simulink model "Pwm_Scalar_control"  (R2021b)
settings: Solver=FixedStepDiscrete  StartTime=0.0  StopTime=inf  RelTol=1e-3  EnableMultiTasking=on
undefined symbols (not defined in the file or in its folder): Down, Up
libraries: c280xlib x4, simulink x3, c2833xlib x1, c2000lib x1
settings Model: Creator=The MathWorks, Inc.  LastModifiedBy=pawan
settings SolverCC: AlgebraicLoopSolver=TrustRegion
settings DataIOCC: LimitDataPoints=on  SaveFormat=Array  SaveOutput=off  SaveTime=off  ReturnWorkspaceOutputs=off
settings OptimizationCC: ExpressionDepthLimit=2147483647  InitFltsAndDblsToZero=on  LifeSpan=inf  MaxStackSize=64  EfficientTunableParamExpr=on
settings DebuggingCC: UnderspecifiedInitializationDetection=Classic  MergeDetectMultiDrivingBlocksExec=none  SignalResolutionControl=TryResolveAllWithWarning  InheritedTsInSrcMsg=none  MultiTaskDSMMsg=warning  MultiTaskCondExecSysMsg=none  FcnCallInpInsideContextMsg=warning  AllowSymbolicDim=off  StateNameClashWarn=warning  SFUnexpectedBacktrackingDiag=warning  SFNoUnconditionalDefaultTransitionDiag=warning  SFExecutionAtInitializationDiag=none  SFMachineParentedDataDiag=warning  ArithmeticOperatorsInVariantConditions=warning
settings HardwareCC: ProdBitPerChar=16  ProdBitPerInt=16  ProdBitPerPointer=32  ProdBitPerSizeT=32  ProdBitPerPtrDiffT=32  ProdLargestAtomicInteger=Integer  ProdLargestAtomicFloat=None  ProdWordSize=16  ProdHWDeviceType=Texas Instruments->C2000  TargetBitPerChar=16  TargetBitPerInt=16  TargetBitPerPointer=16  TargetLargestAtomicInteger=Integer  TargetIntDivRoundTo=Zero  TargetEndianess=LittleEndian  TargetWordSize=16  TargetHWDeviceType=Texas Instruments->C2000  ProdEqTarget=off
settings ModelReferenceCC: PropagateSignalLabelsOutOfModel=off
settings SFSimCC: SimUseLocalCustomCode=off  MATLABDynamicMemAlloc=off  CustomCodeUndefinedFunction=UseInterfaceOnly
settings RTWCC: Description=Embedded Coder  SystemTargetFile=ert.tlc  HardwareBoard=TI Delfino F2833x  TemplateMakefile=ert_default_tmf  PostCodeGenCommand=; codertarget.postCodeGenHookCommand(h)  RTWUseLocalCustomCode=off  Toolchain=Texas Instruments Code Composer Studio (C2000)
settings CodeAppCC: IgnoreCustomStorageClasses=off  CustomSymbolStrType=$N$R$M  StateflowObjectComments=on  InternalIdentifier=Classic
settings ERTTargetCC: MultiwordLength=2048  ParMdlRefBuildCompliant=off  CompOptLevelCompliant=off  ConcurrentExecutionCompliant=off  CPPClassGenCompliant=off  ExtModeTransport=4  ExtModeStaticAlloc=on  ExtModeStaticAllocSize=2048  ExtModeMexFile=ext_xcp  ExtModeIntrfLevel=Level2 - Open  ConvertIfToSwitch=off  SuppressUnreachableDefaultCases=off
settings ConfigComp: CovMetricSettings=dw  CovSaveCumulativeToWorkspaceVar=on  CovSaveSingleToWorkspaceVar=on  CovExternalEMLEnable=off  CovSFcnEnable=off

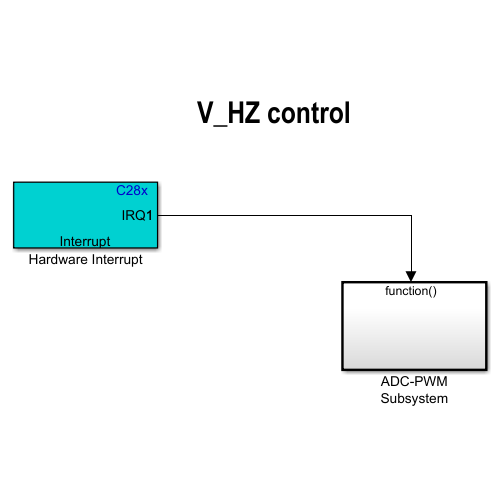
[thumbnail: Simulink's stored preview of the top-level diagram]
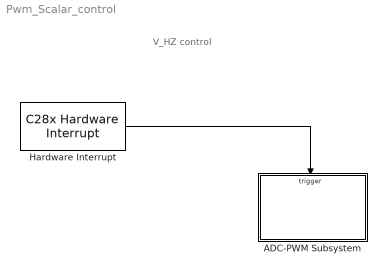
== system Pwm_Scalar_control ==
  note: V_HZ control
  ADC-PWM Subsystem : Subsystem  TreatAsAtomicUnit=on
  Hardware Interrupt : c2000lib/Scheduling/C28x Hardware Interrupt  irqnumbers=[1]  pienumbers=[1]  irqpriorities=[30]  irqpreempts=[0]  showinput=off  dspchiptype=C280X
      settings: SourceProductBaseCode=TIC2000
  wires:
  Hardware Interrupt/1 -> ADC-PWM Subsystem/Trigger

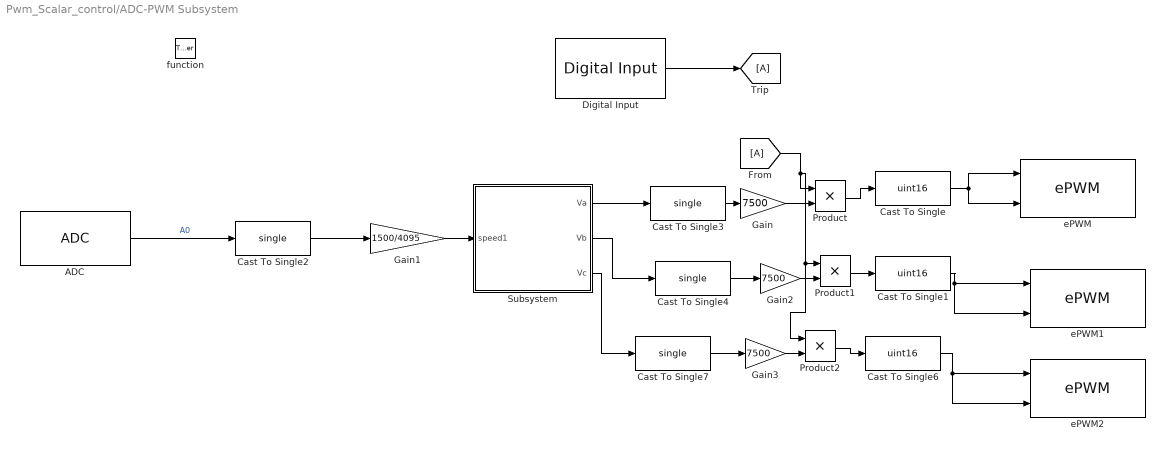
== system Pwm_Scalar_control/ADC-PWM Subsystem ==
  function : TriggerPort  TriggerType=function-call  VariantControl=Variant
  ADC : c280xlib/ADC  useModule=A  useMode=Sequential  sourceSOC=Software  sourceSOC1=ePWMxA  sourceSOC2=ePWMxB  xint2_ADCSOC=31  Ts=-1  dType=single  postInterrupt=on  numConversionsSingle=1  numConversionsDouble=1  conv0=ADCINA0  conv1=ADCINA1  conv2=ADCINA2  conv3=ADCINA3  conv4=ADCINA4  conv5=ADCINA5  conv6=ADCINA6  conv7=ADCINA7  conv8=ADCINB0  conv9=ADCINB1  conv10=ADCINB2  conv11=ADCINB3  conv12=ADCINB4  conv13=ADCINB5  conv14=ADCINB6  conv15=ADCINB7  convAB0=ADCINA0 and ADCINB0  convAB1=ADCINA1 and ADCINB1  convAB2=ADCINA2 and ADCINB2  convAB3=ADCINA3 and ADCINB3  convAB4=ADCINA4 and ADCINB4  convAB5=ADCINA5 and ADCINB5  convAB6=ADCINA6 and ADCINB6  convAB7=ADCINA7 and ADCINB7  convA0=ADCINA0  convA1=ADCINA1  convA2=ADCINA2  convA3=ADCINA3  convA4=ADCINA4  convA5=ADCINA5  convA6=ADCINA6  convA7=ADCINA7  convB0=ADCINB0  convB1=ADCINB1  convB2=ADCINB2  convB3=ADCINB3  convB4=ADCINB4  convB5=ADCINB5  convB6=ADCINB6  convB7=ADCINB7  c28xmultiPort=off  endma=off  chdma=1
      settings: SourceProductBaseCode=TIC2000
  Cast To Single : DataTypeConversion  OutDataTypeStr=uint16
  Cast To Single1 : DataTypeConversion  OutDataTypeStr=uint16
  Cast To Single{2..4,7} (4 alike) : DataTypeConversion  OutDataTypeStr=single  LockScale=on
  Cast To Single6 : DataTypeConversion  OutDataTypeStr=uint16
  Digital Input : c2833xlib/Digital Input  GPIO_Number=GPIO56~GPIO63  GPIO_Bit0=off  GPIO_Bit1=off  GPIO_Bit2=off  GPIO_Bit3=off  GPIO_Bit4=on  GPIO_Bit5=off  GPIO_Bit6=off  GPIO_Bit7=off  sampleTime=-1  dataType=auto  GPIO_Bit0_Qualification=Sync to SYSCLKOUT  GPIO_Bit1_Qualification=Sync to SYSCLKOUT  GPIO_Bit2_Qualification=Sync to SYSCLKOUT  GPIO_Bit3_Qualification=Sync to SYSCLKOUT  GPIO_Bit4_Qualification=Sync to SYSCLKOUT  GPIO_Bit5_Qualification=Sync to SYSCLKOUT  GPIO_Bit6_Qualification=Sync to SYSCLKOUT  GPIO_Bit7_Qualification=Sync to SYSCLKOUT  Qualification_Period=-1
      settings: SourceProductBaseCode=TIC2000
  Gain : Gain  Gain=7500
  Gain1 : Gain  Gain=1500/4095  OutDataTypeStr=Inherit: Same as input  ParamDataTypeStr=Inherit: Same as input
  Gain2 : Gain  Gain=7500
  Gain3 : Gain  Gain=7500
  Product : Product
  Product1 : Product
  Product2 : Product
  Subsystem : Subsystem
  ePWM : c280xlib/ePWM  checkMode=off  useModule=ePWM2  periodUnits=Clock cycles  timerSource=Specify via dialog  timerPeriod_clk=7500  timerPeriod_sec=0.0001  tbshadow=Counter equals to zero  countingMode=Up-Down  phaseActiveEnable=Disable  phaseDirection=Count down after sync  phaseActive=0  synchronizationEnable=off  synchronizationOption=Disable  clockPrescale=1  HSclockPrescale=1  ePWMxAStatus=on  CMPAUnits=Clock cycles  CMPASource=Input port  CMPAValue_per=0  CMPAValue_clk=0  enCMPAshadow=Counter equals to zero  ePWMxAactionLogic1=Do nothing  ePWMxAactionLogic2=Do nothing  ePWMxAactionLogic3=Clear  ePWMxAactionLogic4=Set  ePWMxAactionLogic5=Do nothing  ePWMxAactionLogic6=Do nothing  ePWMxALoadMode=Load on counter equals to zero (CTR=Zero)  ePWMxACSFenable=off  ePWMxACSFvalue=Forcing disable  ePWMxASFreload=Zero  enHRPWM=off  HRPWM_LoadMode=Counter equals to zero (CTR=ZERO)  HRPWM_CTLMode=Phase control mode  HRPWM_EDGMode=Both edge  enSFO=on  ePWMxBStatus=off  CMPBUnits=Percentages  CMPBSource=Input port  CMPBValue_per=0  CMPBValue_clk=0  enCMPBshadow=Counter equals to zero  ePWMxBactionLogic1=Do nothing  ePWMxBactionLogic2=Do nothing  ePWMxBactionLogic3=Do nothing  ePWMxBactionLogic4=Do nothing  ePWMxBactionLogic5=Clear  ePWMxBactionLogic6=Set  ePWMxBLoadMode=Load on counter equals to zero (CTR=Zero)  ePWMxBCSFenable=off  ePWMxBCSFvalue=Forcing disable  ePWMxBSFreload=Zero  enableDBePWMxA=on  enableDBePWMxB=on  DBpolarity=Active high complementary (AHC)  DBedgeDelay=Positive  DBSource_ePWMxA=ePWMxA  DBSource_ePWMxB=ePWMxA  DBperiodSource=Specify via dialog  REDperiod=350  FEDperiod=350  adcstartModuleA=on  adcrequestEventA=First event  adcstartEventA=Counter equals to period (CTR=PRD)  adcstartModuleB=off  adcrequestEventB=First event  adcstartEventB=Counter equals to zero (CTR=Zero)  intEn=off  intPrd=First event  intSel=Counter equals to zero (CTR=Zero)  chopperEnable=off  chopperFrequency=1  chopperFirstwidth=1  chopperDuty=12.5%  tripZonesource=Specify via dialog  tzselOSHT1=off  tzselOSHT2=off  tzselOSHT3=off  tzselOSHT4=off  tzselOSHT5=off  tzselOSHT6=off  tzselCBC1=off  tzselCBC2=off  tzselCBC3=off  tzselCBC4=off  tzselCBC5=off  tzselCBC6=off  enTzOstIntr=off  enTzCbcIntr=off  ePWMxAforced=Low  ePWMxBforced=Low  timerPeriod=-1  ePWMxAValue=1  ePWMxBValue=0  tripZoneoption=One-shot trip (OSHT)
      settings: SourceProductBaseCode=TIC2000
  ePWM1 : c280xlib/ePWM  checkMode=off  useModule=ePWM3  periodUnits=Clock cycles  timerSource=Specify via dialog  timerPeriod_clk=7500  timerPeriod_sec=0.0001  tbshadow=Counter equals to zero  countingMode=Up-Down  phaseActiveEnable=Disable  phaseDirection=Count down after sync  phaseActive=0  synchronizationEnable=off  synchronizationOption=Disable  clockPrescale=1  HSclockPrescale=1  ePWMxAStatus=on  CMPAUnits=Clock cycles  CMPASource=Input port  CMPAValue_per=0  CMPAValue_clk=0  enCMPAshadow=Counter equals to zero  ePWMxAactionLogic1=Do nothing  ePWMxAactionLogic2=Do nothing  ePWMxAactionLogic3=Clear  ePWMxAactionLogic4=Set  ePWMxAactionLogic5=Do nothing  ePWMxAactionLogic6=Do nothing  ePWMxALoadMode=Load on counter equals to zero (CTR=Zero)  ePWMxACSFenable=off  ePWMxACSFvalue=Forcing disable  ePWMxASFreload=Zero  enHRPWM=off  HRPWM_LoadMode=Counter equals to zero (CTR=ZERO)  HRPWM_CTLMode=Phase control mode  HRPWM_EDGMode=Both edge  enSFO=on  ePWMxBStatus=off  CMPBUnits=Percentages  CMPBSource=Input port  CMPBValue_per=0  CMPBValue_clk=0  enCMPBshadow=Counter equals to zero  ePWMxBactionLogic1=Do nothing  ePWMxBactionLogic2=Do nothing  ePWMxBactionLogic3=Do nothing  ePWMxBactionLogic4=Do nothing  ePWMxBactionLogic5=Clear  ePWMxBactionLogic6=Set  ePWMxBLoadMode=Load on counter equals to zero (CTR=Zero)  ePWMxBCSFenable=off  ePWMxBCSFvalue=Forcing disable  ePWMxBSFreload=Zero  enableDBePWMxA=on  enableDBePWMxB=on  DBpolarity=Active high complementary (AHC)  DBedgeDelay=Positive  DBSource_ePWMxA=ePWMxA  DBSource_ePWMxB=ePWMxA  DBperiodSource=Specify via dialog  REDperiod=350  FEDperiod=350  adcstartModuleA=on  adcrequestEventA=First event  adcstartEventA=Counter equals to period (CTR=PRD)  adcstartModuleB=off  adcrequestEventB=First event  adcstartEventB=Counter equals to zero (CTR=Zero)  intEn=off  intPrd=First event  intSel=Counter equals to zero (CTR=Zero)  chopperEnable=off  chopperFrequency=1  chopperFirstwidth=1  chopperDuty=12.5%  tripZonesource=Specify via dialog  tzselOSHT1=off  tzselOSHT2=off  tzselOSHT3=off  tzselOSHT4=off  tzselOSHT5=off  tzselOSHT6=off  tzselCBC1=off  tzselCBC2=off  tzselCBC3=off  tzselCBC4=off  tzselCBC5=off  tzselCBC6=off  enTzOstIntr=off  enTzCbcIntr=off  ePWMxAforced=Low  ePWMxBforced=Low  timerPeriod=-1  ePWMxAValue=1  ePWMxBValue=0  tripZoneoption=One-shot trip (OSHT)
      settings: SourceProductBaseCode=TIC2000
  ePWM2 : c280xlib/ePWM  checkMode=off  useModule=ePWM4  periodUnits=Clock cycles  timerSource=Specify via dialog  timerPeriod_clk=7500  timerPeriod_sec=0.0001  tbshadow=Counter equals to zero  countingMode=Up-Down  phaseActiveEnable=Disable  phaseDirection=Count down after sync  phaseActive=0  synchronizationEnable=off  synchronizationOption=Disable  clockPrescale=1  HSclockPrescale=1  ePWMxAStatus=on  CMPAUnits=Clock cycles  CMPASource=Input port  CMPAValue_per=0  CMPAValue_clk=0  enCMPAshadow=Counter equals to zero  ePWMxAactionLogic1=Do nothing  ePWMxAactionLogic2=Do nothing  ePWMxAactionLogic3=Clear  ePWMxAactionLogic4=Set  ePWMxAactionLogic5=Do nothing  ePWMxAactionLogic6=Do nothing  ePWMxALoadMode=Load on counter equals to zero (CTR=Zero)  ePWMxACSFenable=off  ePWMxACSFvalue=Forcing disable  ePWMxASFreload=Zero  enHRPWM=off  HRPWM_LoadMode=Counter equals to zero (CTR=ZERO)  HRPWM_CTLMode=Phase control mode  HRPWM_EDGMode=Both edge  enSFO=on  ePWMxBStatus=off  CMPBUnits=Percentages  CMPBSource=Input port  CMPBValue_per=0  CMPBValue_clk=0  enCMPBshadow=Counter equals to zero  ePWMxBactionLogic1=Do nothing  ePWMxBactionLogic2=Do nothing  ePWMxBactionLogic3=Do nothing  ePWMxBactionLogic4=Do nothing  ePWMxBactionLogic5=Clear  ePWMxBactionLogic6=Set  ePWMxBLoadMode=Load on counter equals to zero (CTR=Zero)  ePWMxBCSFenable=off  ePWMxBCSFvalue=Forcing disable  ePWMxBSFreload=Zero  enableDBePWMxA=on  enableDBePWMxB=on  DBpolarity=Active high complementary (AHC)  DBedgeDelay=Positive  DBSource_ePWMxA=ePWMxA  DBSource_ePWMxB=ePWMxA  DBperiodSource=Specify via dialog  REDperiod=350  FEDperiod=350  adcstartModuleA=on  adcrequestEventA=First event  adcstartEventA=Counter equals to period (CTR=PRD)  adcstartModuleB=off  adcrequestEventB=First event  adcstartEventB=Counter equals to zero (CTR=Zero)  intEn=off  intPrd=First event  intSel=Counter equals to zero (CTR=Zero)  chopperEnable=off  chopperFrequency=1  chopperFirstwidth=1  chopperDuty=12.5%  tripZonesource=Specify via dialog  tzselOSHT1=off  tzselOSHT2=off  tzselOSHT3=off  tzselOSHT4=off  tzselOSHT5=off  tzselOSHT6=off  tzselCBC1=off  tzselCBC2=off  tzselCBC3=off  tzselCBC4=off  tzselCBC5=off  tzselCBC6=off  enTzOstIntr=off  enTzCbcIntr=off  ePWMxAforced=Low  ePWMxBforced=Low  timerPeriod=-1  ePWMxAValue=1  ePWMxBValue=0  tripZoneoption=One-shot trip (OSHT)
      settings: SourceProductBaseCode=TIC2000
  wires:
  ADC/1 -> Cast To Single2/1  "A0"
  Gain1/1 -> Subsystem/1(speed1)
  Cast To Single2/1 -> Gain1/1
  Cast To Single3/1 -> Gain/1
  Cast To Single/1 -> ePWM/2, ePWM/1
  Cast To Single4/1 -> Gain2/1
  Cast To Single1/1 -> ePWM1/1, ePWM1/2
  Cast To Single7/1 -> Gain3/1
  Cast To Single6/1 -> ePWM2/1, ePWM2/2
  Subsystem/3(Vc) -> Cast To Single7/1
  Subsystem/2(Vb) -> Cast To Single4/1
  Subsystem/1(Va) -> Cast To Single3/1
  Gain/1 -> Product/2
  Product/1 -> Cast To Single/1
  Gain2/1 -> Product1/2
  Product1/1 -> Cast To Single1/1
  Product2/1 -> Cast To Single6/1
  Gain3/1 -> Product2/2
  Digital Input/1 -> [A]
  [A] -> Product2/1, Product1/1, Product/1

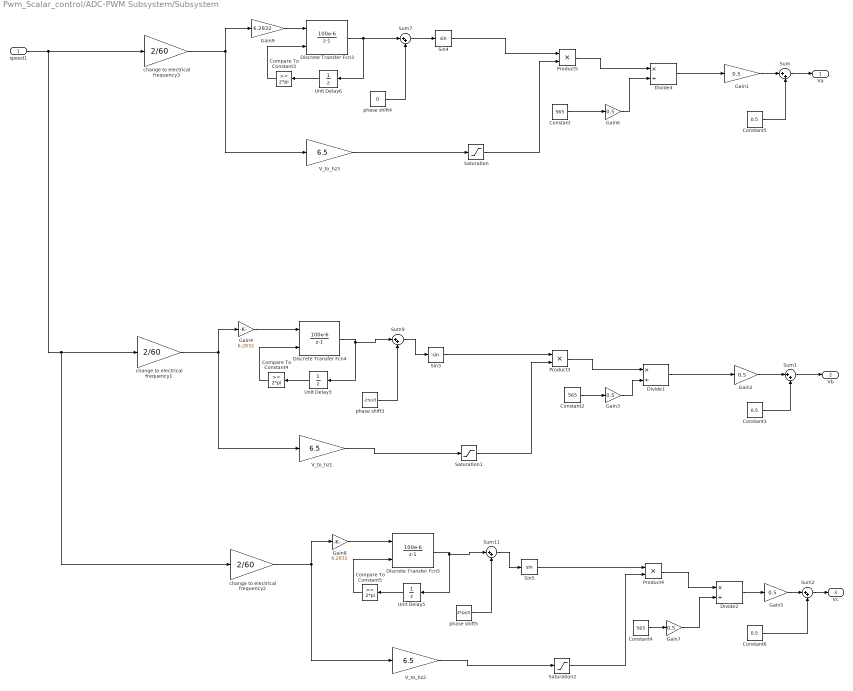
== system Pwm_Scalar_control/ADC-PWM Subsystem/Subsystem ==
  speed1 : Inport
  Compare To Constant3 : simulink/Logic and Bit Operations/Compare To Constant  relop=>=  const=2*pi  OutDataTypeStr=boolean
  Compare To Constant4 : simulink/Logic and Bit Operations/Compare To Constant  relop=>=  const=2*pi  OutDataTypeStr=boolean
  Compare To Constant5 : simulink/Logic and Bit Operations/Compare To Constant  relop=>=  const=2*pi  OutDataTypeStr=boolean
  Constant : Constant  Value=565
  Constant2 : Constant  Value=565
  Constant3 : Constant  Value=0.5  SampleTime=-1
  Constant4 : Constant  Value=565
  Constant5 : Constant  Value=0.5  SampleTime=-1
  Constant6 : Constant  Value=0.5  SampleTime=-1
  Discrete Transfer Fcn3 : DiscreteTransferFcn  Numerator=[100e-6]  Denominator=[1 -1]  ExternalReset=Rising
      settings: InputPortMap=u0,r7
  Discrete Transfer Fcn4 : DiscreteTransferFcn  Numerator=[100e-6]  Denominator=[1 -1]  ExternalReset=Rising
      settings: InputPortMap=u0,r7
  Discrete Transfer Fcn5 : DiscreteTransferFcn  Numerator=[100e-6]  Denominator=[1 -1]  ExternalReset=Rising
      settings: InputPortMap=u0,r7
  Divide1 : Product  Inputs=*/
  Divide2 : Product  Inputs=*/
  Divide4 : Product  Inputs=*/
  Gain{1..3,5..7} (6 alike) : Gain  Gain=0.5
  Gain4 : Gain  Gain=6.2832
  Gain8 : Gain  Gain=6.2832
  Gain9 : Gain  Gain=6.2832
  Product3 : Product
  Product4 : Product
  Product5 : Product
  Saturation : Saturate  UpperLimit=282  LowerLimit=-282
  Saturation1 : Saturate  UpperLimit=282  LowerLimit=-282
  Saturation2 : Saturate  UpperLimit=282  LowerLimit=-282
  Sin3 : Trigonometry
  Sin4 : Trigonometry
  Sin5 : Trigonometry
  Sum{,1..2,7,9,11} (6 alike) : Sum  Inputs=|++
  Unit Delay3 : UnitDelay  SampleTime=-1  HasFrameUpgradeWarning=on
  Unit Delay5 : UnitDelay  SampleTime=-1  HasFrameUpgradeWarning=on
  Unit Delay6 : UnitDelay  SampleTime=-1  HasFrameUpgradeWarning=on
  V_to_hz1 : Gain  Gain=6.5
  V_to_hz2 : Gain  Gain=6.5
  V_to_hz3 : Gain  Gain=6.5
  change to electrical frequency1 : Gain  Gain=2/60
  change to electrical frequency2 : Gain  Gain=2/60
  change to electrical frequency3 : Gain  Gain=2/60
  phase shift3 : Constant  Value=-2*pi/3
  phase shift4 : Constant  Value=0
  phase shift5 : Constant  Value=2*pi/3
  Va : Outport
  Vb : Outport  Port=2
  Vc : Outport  Port=3
  wires:
  change to electrical frequency2/1 -> V_to_hz2/1, Gain8/1
  phase shift5/1 -> Sum11/2
  V_to_hz1/1 -> Saturation1/1
  Sum9/1 -> Sin3/1
  speed1/1 -> change to electrical frequency1/1, change to electrical frequency2/1, change to electrical frequency3/1
  Product3/1 -> Divide1/1
  phase shift3/1 -> Sum9/2
  change to electrical frequency1/1 -> Gain4/1, V_to_hz1/1
  Gain4/1 -> Discrete Transfer Fcn4/1
  Compare To Constant3/1 -> Discrete Transfer Fcn3/2
  Constant2/1 -> Gain3/1
  Discrete Transfer Fcn4/1 -> Unit Delay3/1, Sum9/1
  V_to_hz3/1 -> Saturation/1
  Discrete Transfer Fcn3/1 -> Unit Delay6/1, Sum7/1
  Divide4/1 -> Gain1/1
  Sum7/1 -> Sin4/1
  Constant/1 -> Gain6/1
  Gain6/1 -> Divide4/2
  V_to_hz2/1 -> Saturation2/1
  Unit Delay6/1 -> Compare To Constant3/1
  Divide2/1 -> Gain5/1
  phase shift4/1 -> Sum7/2
  Product4/1 -> Divide2/1
  Compare To Constant4/1 -> Discrete Transfer Fcn4/2
  Gain9/1 -> Discrete Transfer Fcn3/1
  Constant4/1 -> Gain7/1
  Unit Delay3/1 -> Compare To Constant4/1
  Gain7/1 -> Divide2/2
  change to electrical frequency3/1 -> Gain9/1, V_to_hz3/1
  Discrete Transfer Fcn5/1 -> Sum11/1, Unit Delay5/1
  Saturation1/1 -> Product3/2
  Product5/1 -> Divide4/1
  Compare To Constant5/1 -> Discrete Transfer Fcn5/2
  Saturation2/1 -> Product4/2
  Gain3/1 -> Divide1/2
  Unit Delay5/1 -> Compare To Constant5/1
  Divide1/1 -> Gain2/1
  Sum11/1 -> Sin5/1
  Saturation/1 -> Product5/2
  Gain8/1 -> Discrete Transfer Fcn5/1
  Sin4/1 -> Product5/1
  Sin3/1 -> Product3/1
  Sin5/1 -> Product4/1
  Gain1/1 -> Sum/1
  Sum/1 -> Va/1
  Constant5/1 -> Sum/2
  Gain2/1 -> Sum1/1
  Sum1/1 -> Vb/1
  Constant3/1 -> Sum1/2
  Gain5/1 -> Sum2/1
  Sum2/1 -> Vc/1
  Constant6/1 -> Sum2/2
